simulink model "multilevelinverter1"  (R2014a)
settings: Solver=ode23tb  StartTime=0.0  StopTime=1  RelTol=1e-3
undefined symbols (not defined in the file): a, Gn, Ipvn, Iscn, k, Ki, Kv, Npp, Ns, Nss, q, Rp, Rs, Tn, Vocn
libraries: powerlib x102, simulink x34, dsparch4 x12, powerlib_extras x12, powerlib_meascontrol x3
(part 1 of 2)
settings Model: Creator=Muruganandham  LastModifiedBy=selva
settings DataIOCC: SignalLoggingSaveFormat=ModelDataLogs
settings OptimizationCC: ExpressionDepthLimit=2147483647
settings DebuggingCC: UnderspecifiedInitializationDetection=Classic  FcnCallInpInsideContextMsg=UseLocalSettings  StateNameClashWarn=warning
settings GRTTargetCC: CombineOutputUpdateFcns=off  GRTInterface=on

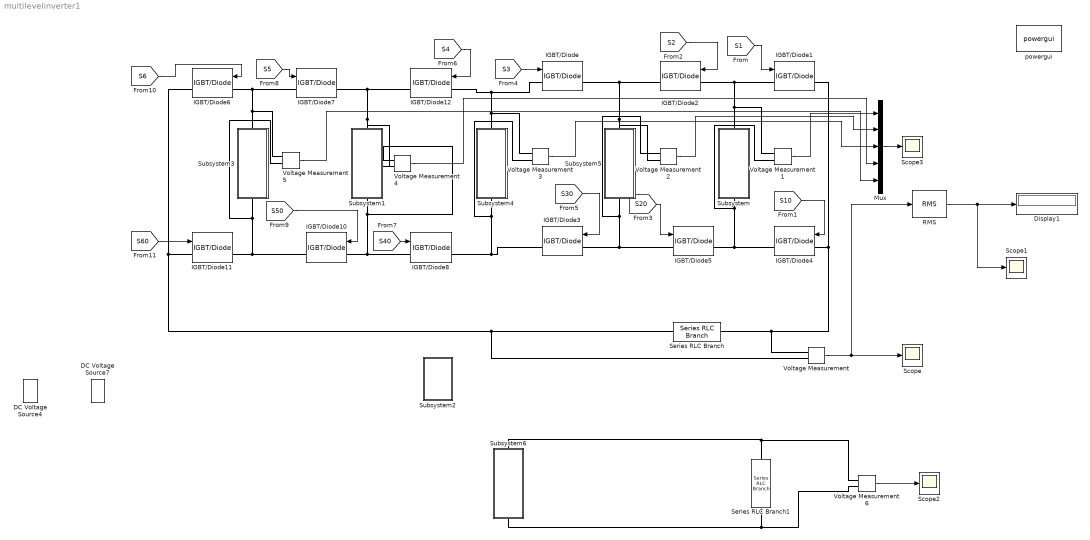
== system multilevelinverter1 ==
  DC Voltage Source4 : powerlib/Electrical Sources/DC Voltage Source  Amplitude=100  Measurements=None
  DC Voltage Source7 : powerlib/Electrical Sources/DC Voltage Source  Amplitude=100  Measurements=None
  Display1 : Display
  IGBT/Diode{,1..8,10..12} (12 alike) : powerlib/Power Electronics/IGBT//Diode  Ron=1e-3  Rs=1e5  Cs=inf  Measurements=on
  Mux : Mux  Inputs=5
  RMS : powerlib_meascontrol/Measurements/RMS  TrueRMS=on  Freq=50  RMSInit=0  Ts=0
  Scope{,1..3} (4 alike) : Scope
      Scope settings: YMin=-300  YMax=300  SaveName=bh
      Scope1 settings: YMin=0  YMax=400  SaveName=bh1
      Scope2 settings: YMin=31.5  YMax=33  SaveName=bh2
      Scope3 settings: YMin=-400  YMax=400  SaveName=bh3
  Series RLC Branch : powerlib/Elements/Series RLC Branch  LConnTagsString=__new0  RConnTagsString=__new0  BranchType=R  Resistance=50  Inductance=1e-3  SetiL0=off  InitialCurrent=0  Capacitance=1e-6  Setx0=off  InitialVoltage=0  Measurements=None
  Series RLC Branch1 : powerlib/Elements/Series RLC Branch  LConnTagsString=__new0  RConnTagsString=__new0  BranchType=R  Resistance=50  Inductance=1e-3  SetiL0=off  InitialCurrent=0  Capacitance=1e-6  Setx0=off  InitialVoltage=0  Measurements=None
  Subsystem : Subsystem
  Subsystem1 : Subsystem
  Subsystem2 : Subsystem  mask{fc=5e3, m=1}
      mask prompts: fc "Switching frequency"; m "modulation index"
  Subsystem3 : Subsystem
  Subsystem4 : Subsystem
  Subsystem5 : Subsystem
  Subsystem6 : Subsystem
  Voltage Measurement{,1..6} (7 alike) : powerlib/Measurements/Voltage Measurement  PhasorSimulation=off  OutputType=Complex  PSBequivalent=0
  powergui : powerlib/powergui  Priority=1  SimulationMode=Discrete  SolverType=Tustin  SampleTime=50e-5  frequency=60  SPID=off  DisableSnubberDevices=off  DisableRonSwitches=off  DisableVfSwitches=off  SwTol=0  Interpol=off  DisplayEquations=off  Ts=0  methode=off  frequencyindice=0  Pbase=100e6  ErrMax=1e-4  Iterations=50  UnitsV=kV  UnitsW=MW  FunctionMessages=off  echomessages=off  HookPort=off  EnableUseOfTLC=off  x0status=blocks  RestoreLinks=warning  ResistiveCurrentMeasurement=off  Frange=[0:2:500]  Ylog=off  Xlog=on  ShowGrid=off  save=off  variable=ZData  structure=bh  ZoomFFT=off  StartTime=0.0  cycles=50  DisplayStyle=1  fundamental=50  FreqAxis=off  MaxFrequency=1000  frequencyindicesteady=1  RmsSteady=1  display=off
  wires:
  [S1] -> IGBT/Diode1/1
  [S10] -> IGBT/Diode4/1
  [S2] -> IGBT/Diode2/1
  [S20] -> IGBT/Diode5/1
  [S3] -> IGBT/Diode/1
  [S30] -> IGBT/Diode3/1
  Voltage Measurement/1 -> RMS/1, Scope/1
  [S40] -> IGBT/Diode8/1
  [S6] -> IGBT/Diode6/1
  [S4] -> IGBT/Diode12/1
  [S5] -> IGBT/Diode7/1
  [S50] -> IGBT/Diode10/1
  [S60] -> IGBT/Diode11/1
  RMS/1 -> Scope1/1, Display1/1
  Voltage Measurement2/1 -> Mux/2
  Voltage Measurement1/1 -> Mux/1
  Voltage Measurement3/1 -> Mux/3
  Voltage Measurement4/1 -> Mux/4
  Voltage Measurement5/1 -> Mux/5
  Mux/1 -> Scope3/1
  Voltage Measurement6/1 -> Scope2/1
  connections:
  IGBT/Diode2/RConn1 -- IGBT/Diode/RConn1 -- Voltage Measurement2/LConn2 -- Subsystem5/RConn1
  IGBT/Diode2/LConn1 -- Voltage Measurement1/LConn1 -- Subsystem/LConn1 -- IGBT/Diode1/LConn1
  IGBT/Diode5/LConn1 -- Voltage Measurement2/LConn1 -- Subsystem5/LConn1 -- IGBT/Diode3/LConn1
  IGBT/Diode5/RConn1 -- Voltage Measurement1/LConn2 -- Subsystem/RConn1 -- IGBT/Diode4/RConn1
  Series RLC Branch/RConn1 -- IGBT/Diode1/RConn1 -- IGBT/Diode4/LConn1 -- Voltage Measurement/LConn1
  IGBT/Diode6/LConn1 -- Voltage Measurement5/LConn1 -- Subsystem3/LConn1 -- IGBT/Diode7/LConn1
  IGBT/Diode7/RConn1 -- Voltage Measurement4/LConn2 -- Subsystem1/RConn1 -- IGBT/Diode12/RConn1
  IGBT/Diode11/RConn1 -- Voltage Measurement5/LConn2 -- Subsystem3/RConn1 -- IGBT/Diode10/RConn1
  IGBT/Diode10/LConn1 -- Voltage Measurement4/LConn1 -- Subsystem1/LConn1 -- IGBT/Diode8/LConn1
  Series RLC Branch/LConn1 -- Voltage Measurement/LConn2 -- IGBT/Diode11/LConn1 -- IGBT/Diode6/RConn1
  IGBT/Diode/LConn1 -- Voltage Measurement3/LConn1 -- Subsystem4/LConn1 -- IGBT/Diode12/LConn1
  IGBT/Diode3/RConn1 -- Voltage Measurement3/LConn2 -- Subsystem4/RConn1 -- IGBT/Diode8/RConn1
  Series RLC Branch1/RConn1 -- Voltage Measurement6/LConn1 -- Subsystem6/LConn1
  Subsystem6/RConn1 -- Voltage Measurement6/LConn2 -- Series RLC Branch1/LConn1

== system multilevelinverter1/Subsystem ==
  Current Measurement : powerlib/Measurements/Current Measurement  PhasorSimulation=off  OutputType=Complex  PSBequivalent=0
  Divide : Product  Inputs=**
  Irradiation [W/m2] 1 : Constant  Value=1000
  Irradiation [W/m2] 2 : Constant
  PV Boost Converter1 : Subsystem
  PV model subsystem1 : Subsystem
  Temperature [K]1 : Constant  Value=25+273.15
  + : PMIOPort  Port=1  Side=Left
  - : PMIOPort  Port=2  Side=Right
  wires:
  Temperature [K]1/1 -> PV model subsystem1/1(T)
  Divide/1 -> PV model subsystem1/2(G)
  Irradiation [W/m2] 1/1 -> Divide/1
  Irradiation [W/m2] 2/1 -> Divide/2
  connections:
  PV Boost Converter1/LConn2 -- PV model subsystem1/RConn2
  Current Measurement/LConn1 -- PV model subsystem1/RConn1
  PV Boost Converter1/LConn1 -- Current Measurement/RConn1
  PV Boost Converter1/RConn1 -- +/RConn1
  PV Boost Converter1/RConn2 -- -/RConn1

== system multilevelinverter1/Subsystem1 ==
  Current Measurement : powerlib/Measurements/Current Measurement  PhasorSimulation=off  OutputType=Complex  PSBequivalent=0
  Divide : Product  Inputs=**
  Irradiation [W/m2] 1 : Constant  Value=1000
  Irradiation [W/m2] 2 : Constant
  PV Boost Converter1 : Subsystem
  PV model subsystem1 : Subsystem
  Temperature [K]1 : Constant  Value=25+273.15
  + : PMIOPort  Port=1  Side=Left
  - : PMIOPort  Port=2  Side=Right
  wires:
  Irradiation [W/m2] 2/1 -> Divide/2
  Irradiation [W/m2] 1/1 -> Divide/1
  Divide/1 -> PV model subsystem1/2(G)
  Temperature [K]1/1 -> PV model subsystem1/1(T)
  connections:
  PV Boost Converter1/RConn2 -- -/RConn1
  PV Boost Converter1/RConn1 -- +/RConn1
  PV Boost Converter1/LConn1 -- Current Measurement/RConn1
  Current Measurement/LConn1 -- PV model subsystem1/RConn1
  PV Boost Converter1/LConn2 -- PV model subsystem1/RConn2

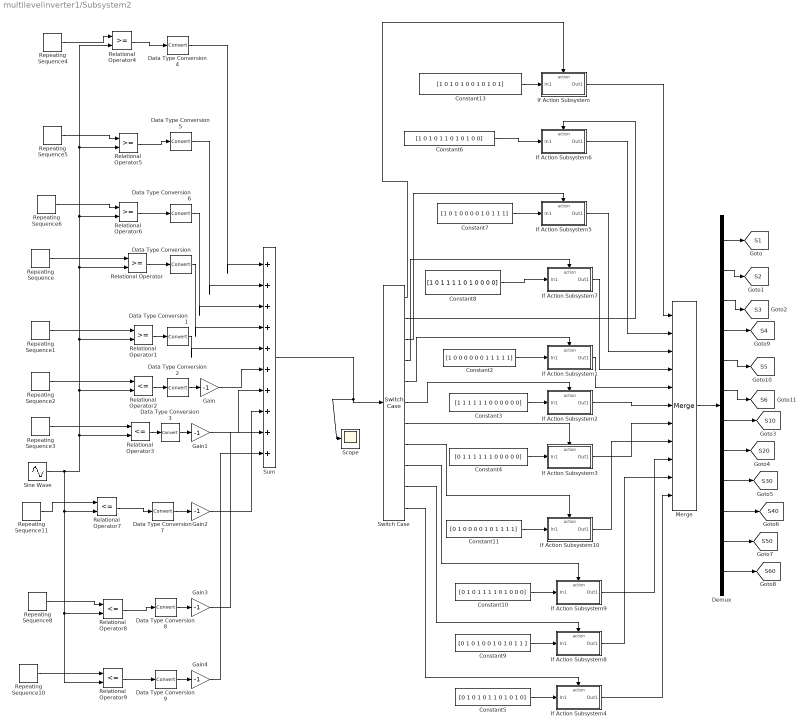
== system multilevelinverter1/Subsystem2 ==
  Constant10 : Constant  Value=[0 1 0 1 1 1 1 0 1 0 0 0]
  Constant11 : Constant  Value=[0 1 0 0 0 0 1 0 1 1 1 1]
  Constant13 : Constant  Value=[1 0 1 0 1 0 0 1 0 1 0 1]
  Constant2 : Constant  Value=[1 0 0 0 0 0 0 1 1 1 1 1]
  Constant3 : Constant  Value=[1 1 1 1 1 1 0 0 0 0 0 0]
  Constant4 : Constant  Value=[0 1 1 1 1 1 1 0 0 0 0 0]
  Constant5 : Constant  Value=[0 1 0 1 0 1 1 0 1 0 1 0]
  Constant6 : Constant  Value=[1 0 1 0 1 1 0 1 0 1 0 0]
  Constant7 : Constant  Value=[1 0 1 0 0 0 0 1 0 1 1 1]
  Constant8 : Constant  Value=[1 0 1 1 1 1 0 1 0 0 0 0]
  Constant9 : Constant  Value=[0 1 0 1 0 0 1 0 1 0 1 1 ]
  Data Type Conversion{,1..9} (10 alike) : DataTypeConversion
  Demux : Demux  Outputs=12
  Gain{,1..4} (5 alike) : Gain  Gain=-1
  If Action Subsystem : Subsystem  TreatAsAtomicUnit=on
  If Action Subsystem1 : Subsystem  TreatAsAtomicUnit=on
  If Action Subsystem10 : Subsystem  TreatAsAtomicUnit=on
  If Action Subsystem2 : Subsystem  TreatAsAtomicUnit=on
  If Action Subsystem3 : Subsystem  TreatAsAtomicUnit=on
  If Action Subsystem4 : Subsystem  TreatAsAtomicUnit=on
  If Action Subsystem5 : Subsystem  TreatAsAtomicUnit=on
  If Action Subsystem6 : Subsystem  TreatAsAtomicUnit=on
  If Action Subsystem7 : Subsystem  TreatAsAtomicUnit=on
  If Action Subsystem8 : Subsystem  TreatAsAtomicUnit=on
  If Action Subsystem9 : Subsystem  TreatAsAtomicUnit=on
  Merge : Merge  Inputs=11
  Relational Operator{,1,4..6} (5 alike) : RelationalOperator  OutDataTypeStr=boolean
  Relational Operator{2..3,7..9} (5 alike) : RelationalOperator  Operator=<=  OutDataTypeStr=boolean
  Repeating Sequence : simulink/Sources/Repeating Sequence  rep_seq_t="[0 (1/fc)/2  (1/fc)]"  rep_seq_y=[2 1 2]
  Repeating Sequence1 : simulink/Sources/Repeating Sequence  rep_seq_t="[0 (1/fc)/2  (1/fc)]"  rep_seq_y=[1 0 1]
  Repeating Sequence10 : simulink/Sources/Repeating Sequence  rep_seq_t="[0 (1/fc)/2  (1/fc)]"  rep_seq_y=[-5 -4 -5]
  Repeating Sequence11 : simulink/Sources/Repeating Sequence  rep_seq_t="[0 (1/fc)/2  (1/fc)]"  rep_seq_y=[-3 -2 -3]
  Repeating Sequence2 : simulink/Sources/Repeating Sequence  rep_seq_t="[0 (1/fc)/2  (1/fc)]"  rep_seq_y=[-1 0 -1]
  Repeating Sequence3 : simulink/Sources/Repeating Sequence  rep_seq_t="[0 (1/fc)/2  (1/fc)]"  rep_seq_y=[-2 -1 -2]
  Repeating Sequence4 : simulink/Sources/Repeating Sequence  rep_seq_t="[0 (1/fc)/2  (1/fc)]"  rep_seq_y=[4 5 4]
  Repeating Sequence5 : simulink/Sources/Repeating Sequence  rep_seq_t="[0 (1/fc)/2  (1/fc)]"  rep_seq_y=[4 3 4]
  Repeating Sequence6 : simulink/Sources/Repeating Sequence  rep_seq_t="[0 (1/fc)/2  (1/fc)]"  rep_seq_y=[3 2 3]
  Repeating Sequence8 : simulink/Sources/Repeating Sequence  rep_seq_t="[0 (1/fc)/2  (1/fc)]"  rep_seq_y=[-4 -3 -4]
  Scope : Scope
  Sine Wave : Sin  Amplitude=6*m  Frequency=2*pi*50  SampleTime=0
  Sum : Sum  Inputs=|++++++++++
  Switch Case : SwitchCase  CaseConditions={-5, -4, -3, -2, -1, 0, 1, 2, 3, 4, 5}  ShowDefaultCase=off
  tag scope: S10=global, S1=global, S20=global, S2=global, S30=global, S3=global, S40=global, S4=global, S50=global, S5=global, S60=global, S6=global
  wires:
  Data Type Conversion3/1 -> Gain1/1
  Data Type Conversion2/1 -> Gain/1
  Relational Operator3/1 -> Data Type Conversion3/1
  Relational Operator2/1 -> Data Type Conversion2/1
  Repeating Sequence3/1 -> Relational Operator3/1
  Repeating Sequence2/1 -> Relational Operator2/1
  Repeating Sequence1/1 -> Relational Operator1/1
  Repeating Sequence/1 -> Relational Operator/1
  Relational Operator1/1 -> Data Type Conversion1/1
  Relational Operator/1 -> Data Type Conversion/1
  Merge/1 -> Demux/1
  If Action Subsystem/1(Out1) -> Merge/1
  Constant4/1 -> If Action Subsystem3/1(In1)
  Constant3/1 -> If Action Subsystem2/1(In1)
  Constant2/1 -> If Action Subsystem1/1(In1)
  Repeating Sequence6/1 -> Relational Operator6/1
  Repeating Sequence5/1 -> Relational Operator5/1
  Repeating Sequence4/1 -> Relational Operator4/1
  Relational Operator6/1 -> Data Type Conversion6/1
  Relational Operator5/1 -> Data Type Conversion5/1
  Relational Operator4/1 -> Data Type Conversion4/1
  Repeating Sequence8/1 -> Relational Operator8/1
  Repeating Sequence11/1 -> Relational Operator7/1
  Sine Wave/1 -> Relational Operator9/2, Relational Operator8/2, Relational Operator7/2, Relational Operator3/2, Relational Operator2/2, Relational Operator6/2, Relational Operator5/2, Relational Operator4/2, Relational Operator/2, Relational Operator1/2
  Relational Operator9/1 -> Data Type Conversion9/1
  Relational Operator8/1 -> Data Type Conversion8/1
  Relational Operator7/1 -> Data Type Conversion7/1
  Data Type Conversion9/1 -> Gain4/1
  Data Type Conversion8/1 -> Gain3/1
  Data Type Conversion7/1 -> Gain2/1
  Repeating Sequence10/1 -> Relational Operator9/1
  Data Type Conversion4/1 -> Sum/1
  Data Type Conversion5/1 -> Sum/2
  Data Type Conversion6/1 -> Sum/3
  Data Type Conversion/1 -> Sum/4
  Data Type Conversion1/1 -> Sum/5
  Gain/1 -> Sum/6
  Gain1/1 -> Sum/7
  Gain2/1 -> Sum/8
  Gain3/1 -> Sum/9
  Gain4/1 -> Sum/10
  Switch Case/6 -> If Action Subsystem2/Action
  If Action Subsystem6/1(Out1) -> Merge/2
  If Action Subsystem5/1(Out1) -> Merge/3
  If Action Subsystem7/1(Out1) -> Merge/4
  If Action Subsystem1/1(Out1) -> Merge/5
  If Action Subsystem2/1(Out1) -> Merge/6
  If Action Subsystem3/1(Out1) -> Merge/7
  Constant9/1 -> If Action Subsystem8/1(In1)
  Constant10/1 -> If Action Subsystem9/1(In1)
  Constant11/1 -> If Action Subsystem10/1(In1)
  Switch Case/11 -> If Action Subsystem4/Action
  If Action Subsystem4/1(Out1) -> Merge/11
  Switch Case/10 -> If Action Subsystem8/Action
  Switch Case/9 -> If Action Subsystem9/Action
  Switch Case/8 -> If Action Subsystem10/Action
  Switch Case/7 -> If Action Subsystem3/Action
  Switch Case/5 -> If Action Subsystem1/Action
  Switch Case/4 -> If Action Subsystem7/Action
  Switch Case/3 -> If Action Subsystem5/Action
  Switch Case/2 -> If Action Subsystem6/Action
  Switch Case/1 -> If Action Subsystem/Action
  Constant6/1 -> If Action Subsystem6/1(In1)
  Constant7/1 -> If Action Subsystem5/1(In1)
  Constant8/1 -> If Action Subsystem7/1(In1)
  If Action Subsystem10/1(Out1) -> Merge/8
  If Action Subsystem9/1(Out1) -> Merge/9
  If Action Subsystem8/1(Out1) -> Merge/10
  Demux/3 -> [S3]
  Demux/2 -> [S2]
  Demux/1 -> [S1]
  Demux/7 -> [S10]
  Demux/8 -> [S20]
  Demux/9 -> [S30]
  Demux/10 -> [S40]
  Demux/11 -> [S50]
  Demux/12 -> [S60]
  Demux/6 -> [S6]
  Demux/5 -> [S5]
  Demux/4 -> [S4]
  Sum/1 -> Scope/1, Switch Case/1
  Constant5/1 -> If Action Subsystem4/1(In1)
  Constant13/1 -> If Action Subsystem/1(In1)

== system multilevelinverter1/Subsystem3 ==
  Current Measurement : powerlib/Measurements/Current Measurement  PhasorSimulation=off  OutputType=Complex  PSBequivalent=0
  Divide : Product  Inputs=**
  Irradiation [W/m2] 1 : Constant  Value=1000
  Irradiation [W/m2] 2 : Constant
  PV Boost Converter1 : Subsystem
  PV model subsystem1 : Subsystem
  Temperature [K]1 : Constant  Value=25+273.15
  + : PMIOPort  Port=1  Side=Left
  - : PMIOPort  Port=2  Side=Right
  wires:
  Irradiation [W/m2] 2/1 -> Divide/2
  Irradiation [W/m2] 1/1 -> Divide/1
  Divide/1 -> PV model subsystem1/2(G)
  Temperature [K]1/1 -> PV model subsystem1/1(T)
  connections:
  PV Boost Converter1/RConn2 -- -/RConn1
  PV Boost Converter1/RConn1 -- +/RConn1
  PV Boost Converter1/LConn1 -- Current Measurement/RConn1
  Current Measurement/LConn1 -- PV model subsystem1/RConn1
  PV Boost Converter1/LConn2 -- PV model subsystem1/RConn2

== system multilevelinverter1/Subsystem4 ==
  Current Measurement : powerlib/Measurements/Current Measurement  PhasorSimulation=off  OutputType=Complex  PSBequivalent=0
  Divide : Product  Inputs=**
  Irradiation [W/m2] 1 : Constant  Value=1000
  Irradiation [W/m2] 2 : Constant
  PV Boost Converter1 : Subsystem
  PV model subsystem1 : Subsystem
  Temperature [K]1 : Constant  Value=25+273.15
  + : PMIOPort  Port=1  Side=Left
  - : PMIOPort  Port=2  Side=Right
  wires:
  Irradiation [W/m2] 2/1 -> Divide/2
  Irradiation [W/m2] 1/1 -> Divide/1
  Divide/1 -> PV model subsystem1/2(G)
  Temperature [K]1/1 -> PV model subsystem1/1(T)
  connections:
  PV Boost Converter1/RConn2 -- -/RConn1
  PV Boost Converter1/RConn1 -- +/RConn1
  PV Boost Converter1/LConn1 -- Current Measurement/RConn1
  Current Measurement/LConn1 -- PV model subsystem1/RConn1
  PV Boost Converter1/LConn2 -- PV model subsystem1/RConn2

== system multilevelinverter1/Subsystem5 ==
  Current Measurement : powerlib/Measurements/Current Measurement  PhasorSimulation=off  OutputType=Complex  PSBequivalent=0
  Divide : Product  Inputs=**
  Irradiation [W/m2] 1 : Constant  Value=1000
  Irradiation [W/m2] 2 : Constant
  PV Boost Converter1 : Subsystem
  PV model subsystem1 : Subsystem
  Temperature [K]1 : Constant  Value=25+273.15
  + : PMIOPort  Port=1  Side=Left
  - : PMIOPort  Port=2  Side=Right
  wires:
  Temperature [K]1/1 -> PV model subsystem1/1(T)
  Divide/1 -> PV model subsystem1/2(G)
  Irradiation [W/m2] 1/1 -> Divide/1
  Irradiation [W/m2] 2/1 -> Divide/2
  connections:
  PV Boost Converter1/LConn2 -- PV model subsystem1/RConn2
  Current Measurement/LConn1 -- PV model subsystem1/RConn1
  PV Boost Converter1/LConn1 -- Current Measurement/RConn1
  PV Boost Converter1/RConn1 -- +/RConn1
  PV Boost Converter1/RConn2 -- -/RConn1

== system multilevelinverter1/Subsystem6 ==
  Current Measurement : powerlib/Measurements/Current Measurement  PhasorSimulation=off  OutputType=Complex  PSBequivalent=0
  Divide : Product  Inputs=**
  Irradiation [W/m2] 1 : Constant  Value=1000
  Irradiation [W/m2] 2 : Constant
  PV Boost Converter1 : Subsystem
  PV model subsystem1 : Subsystem
  Temperature [K]1 : Constant  Value=25+273.15
  + : PMIOPort  Port=1  Side=Left
  - : PMIOPort  Port=2  Side=Right
  wires:
  Temperature [K]1/1 -> PV model subsystem1/1(T)
  Divide/1 -> PV model subsystem1/2(G)
  Irradiation [W/m2] 1/1 -> Divide/1
  Irradiation [W/m2] 2/1 -> Divide/2
  connections:
  PV Boost Converter1/LConn2 -- PV model subsystem1/RConn2
  Current Measurement/LConn1 -- PV model subsystem1/RConn1
  PV Boost Converter1/LConn1 -- Current Measurement/RConn1
  PV Boost Converter1/RConn1 -- +/RConn1
  PV Boost Converter1/RConn2 -- -/RConn1

== system multilevelinverter1/Subsystem/PV Boost Converter1 ==
  Analog Filter Design : dsparch4/Analog Filter Design  method=Butterworth  filttype=Lowpass  N=8  Wlo=30  Whi=80  Rp=2  Rs=40
  Analog Filter Design1 : dsparch4/Analog Filter Design  method=Butterworth  filttype=Lowpass  N=8  Wlo=30  Whi=80  Rp=2  Rs=40
  Current Measurement : powerlib/Measurements/Current Measurement  PhasorSimulation=off  OutputType=Complex  PSBequivalent=0
  Diode : powerlib/Power Electronics/Diode  Ron=0.001  Lon=0  Vf=0.8  IC=0  UseSnubber=off  Rs=500  Cs=250e-9  Measurements=on
  MPPT : Subsystem
  Mosfet : powerlib/Power Electronics/Mosfet  Ron=0.1  Lon=0  Rd=0.01  Vfd=0  IC=0  Rs=1e5  Cs=inf  Measurements=on
  PI CONTOLER : Subsystem
  Relational Operator1 : RelationalOperator  Operator=<=  OutDataTypeStr=boolean
  Repeating Sequence : simulink/Sources/Repeating Sequence  rep_seq_t=[0 0.0001 0.0002]  rep_seq_y=[0 10 0]
  Scope{1..3,8} (4 alike) : Scope
      Scope1 settings: SaveName=ScopeData2
      Scope2 settings: SaveName=ScopeData3
      Scope3 settings: YMin=-20  YMax=100  SaveName=ScopeData12
      Scope8 settings: YMin=31.943  YMax=31.943  SaveName=ScopeData4
  Series RLC Branch : powerlib/Elements/Series RLC Branch  LConnTagsString=__new0  RConnTagsString=__new0  BranchType=L  Resistance=1  Inductance=1e-3  SetiL0=off  InitialCurrent=0  Capacitance=1e-6  Setx0=off  InitialVoltage=0  Measurements=None
  Series RLC Branch1 : powerlib/Elements/Series RLC Branch  LConnTagsString=__new0  RConnTagsString=__new0  BranchType=C  Resistance=1  Inductance=12e-3  SetiL0=off  InitialCurrent=0  Capacitance=2200e-6  Setx0=off  InitialVoltage=0  Measurements=None
  Voltage Measurement1 : powerlib/Measurements/Voltage Measurement  PhasorSimulation=off  OutputType=Complex  PSBequivalent=0
  Voltage Measurement2 : powerlib/Measurements/Voltage Measurement  PhasorSimulation=off  OutputType=Complex  PSBequivalent=0
  + : PMIOPort  Port=1  Side=Right
  - : PMIOPort  Port=2  Side=Right
  Vpv+ : PMIOPort  Tag=PMCPort  Port=3  Side=Left
  Vpv- : PMIOPort  Tag=PMCPort  Port=4  Side=Left
  wires:
  Analog Filter Design1/1 -> MPPT/1(V)
  Analog Filter Design/1 -> MPPT/2(I)
  MPPT/1(D) -> Relational Operator1/2
  Relational Operator1/1 -> Scope1/1
  Repeating Sequence/1 -> Scope2/1, Relational Operator1/1
  Current Measurement/1 -> Analog Filter Design/1
  Voltage Measurement1/1 -> Scope8/1, [A1]
  [A1] -> PI CONTOLER/1(In1)
  PI CONTOLER/1(Out1) -> [G]
  Voltage Measurement2/1 -> Scope3/1, Analog Filter Design1/1
  [G] -> Mosfet/1
  connections:
  Current Measurement/LConn1 -- Vpv+/RConn1
  Diode/RConn1 -- Voltage Measurement1/LConn1 -- +/RConn1 -- Series RLC Branch1/LConn1
  Series RLC Branch/LConn1 -- Current Measurement/RConn1 -- Voltage Measurement2/LConn1
  Series RLC Branch1/RConn1 -- Voltage Measurement1/LConn2 -- -/RConn1 -- Mosfet/RConn1 -- Voltage Measurement2/LConn2 -- Vpv-/RConn1
  Diode/LConn1 -- Mosfet/LConn1 -- Series RLC Branch/RConn1

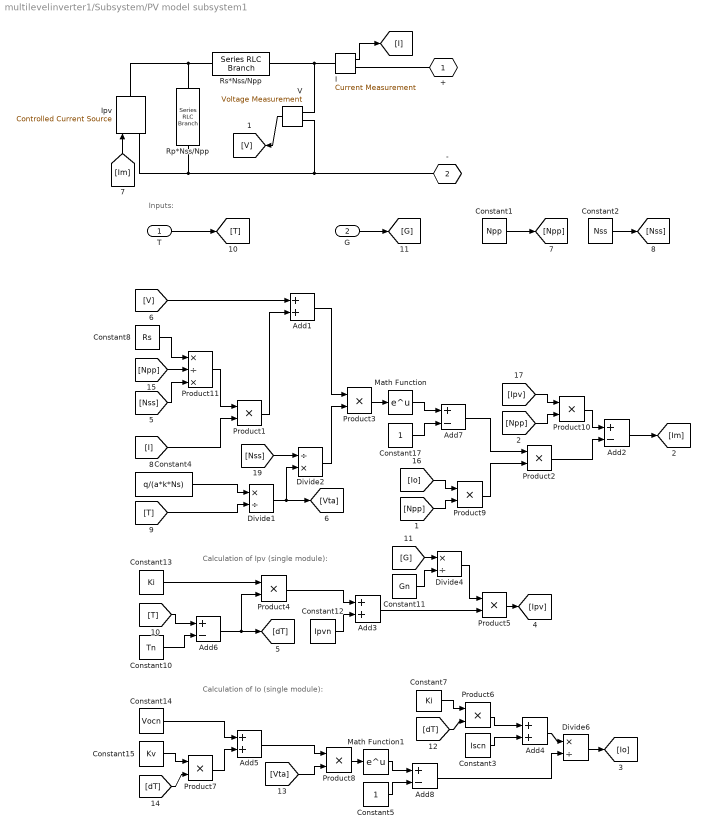
== system multilevelinverter1/Subsystem/PV model subsystem1 ==
  note: Inputs:
  note: Calculation of Ipv (single module):
  note: Calculation of Io (single module):
  T : Inport
  G : Inport  Port=2
  Add{1,3..5} (4 alike) : Sum
  Add{2,6..8} (4 alike) : Sum  Inputs=+-
  Constant1 : Constant  Value=Npp
  Constant10 : Constant  Value=Tn
  Constant11 : Constant  Value=Gn
  Constant12 : Constant  Value=Ipvn
  Constant13 : Constant  Value=Ki
  Constant14 : Constant  Value=Vocn
  Constant15 : Constant  Value=Kv
  Constant17 : Constant
  Constant2 : Constant  Value=Nss
  Constant3 : Constant  Value=Iscn
  Constant4 : Constant  Value=q/(a*k*Ns)
  Constant5 : Constant
  Constant7 : Constant  Value=Ki
  Constant8 : Constant  Value=Rs
  Divide1 : Product  Inputs=*/
  Divide2 : Product  Inputs=/*
  Divide4 : Product  Inputs=*/
  Divide6 : Product  Inputs=*/
  I : powerlib/Measurements/Current Measurement  PhasorSimulation=off  OutputType=Complex  PSBequivalent=0
  Ipv : powerlib/Electrical Sources/Controlled Current Source  Initialize=on  Source_Type=DC  Amplitude=00  Phase=0  Frequency=0  Measurements=None
  Math Function : Math  SaturateOnIntegerOverflow=on
  Math Function1 : Math  SaturateOnIntegerOverflow=on
  Product{1..10} (10 alike) : Product  RndMeth=Zero
  Product11 : Product  Inputs=*/*  RndMeth=Zero
  Rp*Nss/Npp : powerlib/Elements/Series RLC Branch  LConnTagsString=__new0  RConnTagsString=__new0  BranchType=R  Resistance=Rp*Nss/Npp  Inductance=1e-3  SetiL0=off  InitialCurrent=0  Capacitance=1e-6  Setx0=off  InitialVoltage=0  Measurements=None
  Rs*Nss/Npp : powerlib/Elements/Series RLC Branch  LConnTagsString=__new0  RConnTagsString=__new0  BranchType=R  Resistance=Rs*Nss/Npp  Inductance=1e-3  SetiL0=off  InitialCurrent=0  Capacitance=1e-6  Setx0=off  InitialVoltage=0  Measurements=None
  "V " : powerlib/Measurements/Voltage Measurement  PhasorSimulation=off  OutputType=Complex  PSBequivalent=0
  + : PMIOPort  Port=1  Side=Right
  - : PMIOPort  Port=2  Side=Right
  wires:
  I/1 -> [I]
  "V "/1 -> [V]
  [Im] -> Ipv/1
  G/1 -> [G]
  T/1 -> [T]
  Constant10/1 -> Add6/2
  [T] -> Add6/1
  [I] -> Product1/2
  Constant4/1 -> Divide1/1
  [T] -> Divide1/2
  [V] -> Add1/1
  Product3/1 -> Math Function/1
  Add2/1 -> [Im]
  Add1/1 -> Product3/1
  [G] -> Divide4/1
  Constant11/1 -> Divide4/2
  Constant13/1 -> Product4/1
  [dT] -> Product6/2
  Constant7/1 -> Product6/1
  [dT] -> Product7/2
  Constant14/1 -> Add5/1
  Product8/1 -> Math Function1/1
  Add5/1 -> Product8/1
  Constant17/1 -> Add7/2
  Add7/1 -> Product2/1
  Constant5/1 -> Add8/2
  Math Function1/1 -> Add8/1
  Divide6/1 -> [Io]
  Product5/1 -> [Ipv]
  Product1/1 -> Add1/2
  Math Function/1 -> Add7/1
  Product4/1 -> Add3/1
  Add3/1 -> Product5/2
  Divide4/1 -> Product5/1
  Product7/1 -> Add5/2
  Constant15/1 -> Product7/1
  [Vta] -> Product8/2
  Add8/1 -> Divide6/2
  Constant3/1 -> Add4/2
  Product6/1 -> Add4/1
  Constant12/1 -> Add3/2
  Product2/1 -> Add2/2
  Product9/1 -> Product2/2
  [Io] -> Product9/1
  [Npp] -> Product9/2
  Constant1/1 -> [Npp]
  Constant2/1 -> [Nss]
  [Ipv] -> Product10/1
  [Npp] -> Product10/2
  Product10/1 -> Add2/1
  Constant8/1 -> Product11/1
  [Npp] -> Product11/2
  [Nss] -> Product11/3
  Product11/1 -> Product1/1
  [Nss] -> Divide2/1
  Divide1/1 -> Divide2/2, [Vta]
  Divide2/1 -> Product3/2
  Add6/1 -> [dT], Product4/2
  Add4/1 -> Divide6/1
  connections:
  I/LConn1 -- "V "/LConn1 -- Rs*Nss/Npp/RConn1
  -/RConn1 -- Rp*Nss/Npp/RConn1 -- Ipv/LConn1 -- "V "/LConn2
  Ipv/RConn1 -- Rs*Nss/Npp/LConn1 -- Rp*Nss/Npp/LConn1
  +/RConn1 -- I/RConn1

== system multilevelinverter1/Subsystem1/PV Boost Converter1 ==
  Analog Filter Design : dsparch4/Analog Filter Design  method=Butterworth  filttype=Lowpass  N=8  Wlo=30  Whi=80  Rp=2  Rs=40
  Analog Filter Design1 : dsparch4/Analog Filter Design  method=Butterworth  filttype=Lowpass  N=8  Wlo=30  Whi=80  Rp=2  Rs=40
  Current Measurement : powerlib/Measurements/Current Measurement  PhasorSimulation=off  OutputType=Complex  PSBequivalent=0
  Diode : powerlib/Power Electronics/Diode  Ron=0.001  Lon=0  Vf=0.8  IC=0  UseSnubber=off  Rs=500  Cs=250e-9  Measurements=on
  MPPT : Subsystem
  Mosfet : powerlib/Power Electronics/Mosfet  Ron=0.1  Lon=0  Rd=0.01  Vfd=0  IC=0  Rs=1e5  Cs=inf  Measurements=on
  PI CONTOLER : Subsystem
  Relational Operator1 : RelationalOperator  Operator=<=  OutDataTypeStr=boolean
  Repeating Sequence : simulink/Sources/Repeating Sequence  rep_seq_t=[0 0.0001 0.0002]  rep_seq_y=[0 10 0]
  Scope{1..3,8} (4 alike) : Scope
      Scope1 settings: SaveName=ScopeData2
      Scope2 settings: SaveName=ScopeData3
      Scope3 settings: YMin=-20  YMax=100  SaveName=ScopeData12
      Scope8 settings: YMin=31.943  YMax=31.943  SaveName=ScopeData4
  Series RLC Branch : powerlib/Elements/Series RLC Branch  LConnTagsString=__new0  RConnTagsString=__new0  BranchType=L  Resistance=1  Inductance=1e-3  SetiL0=off  InitialCurrent=0  Capacitance=1e-6  Setx0=off  InitialVoltage=0  Measurements=None
  Series RLC Branch1 : powerlib/Elements/Series RLC Branch  LConnTagsString=__new0  RConnTagsString=__new0  BranchType=C  Resistance=1  Inductance=12e-3  SetiL0=off  InitialCurrent=0  Capacitance=2200e-6  Setx0=off  InitialVoltage=0  Measurements=None
  Voltage Measurement1 : powerlib/Measurements/Voltage Measurement  PhasorSimulation=off  OutputType=Complex  PSBequivalent=0
  Voltage Measurement2 : powerlib/Measurements/Voltage Measurement  PhasorSimulation=off  OutputType=Complex  PSBequivalent=0
  + : PMIOPort  Port=1  Side=Right
  - : PMIOPort  Port=2  Side=Right
  Vpv+ : PMIOPort  Tag=PMCPort  Port=3  Side=Left
  Vpv- : PMIOPort  Tag=PMCPort  Port=4  Side=Left
  wires:
  [G] -> Mosfet/1
  Voltage Measurement2/1 -> Analog Filter Design1/1, Scope3/1
  PI CONTOLER/1(Out1) -> [G]
  [A1] -> PI CONTOLER/1(In1)
  Voltage Measurement1/1 -> [A1], Scope8/1
  Current Measurement/1 -> Analog Filter Design/1
  Repeating Sequence/1 -> Relational Operator1/1, Scope2/1
  Relational Operator1/1 -> Scope1/1
  MPPT/1(D) -> Relational Operator1/2
  Analog Filter Design/1 -> MPPT/2(I)
  Analog Filter Design1/1 -> MPPT/1(V)
  connections:
  Series RLC Branch/RConn1 -- Mosfet/LConn1 -- Diode/LConn1
  Vpv-/RConn1 -- Voltage Measurement2/LConn2 -- Mosfet/RConn1 -- -/RConn1 -- Voltage Measurement1/LConn2 -- Series RLC Branch1/RConn1
  Voltage Measurement2/LConn1 -- Current Measurement/RConn1 -- Series RLC Branch/LConn1
  Series RLC Branch1/LConn1 -- +/RConn1 -- Voltage Measurement1/LConn1 -- Diode/RConn1
  Current Measurement/LConn1 -- Vpv+/RConn1

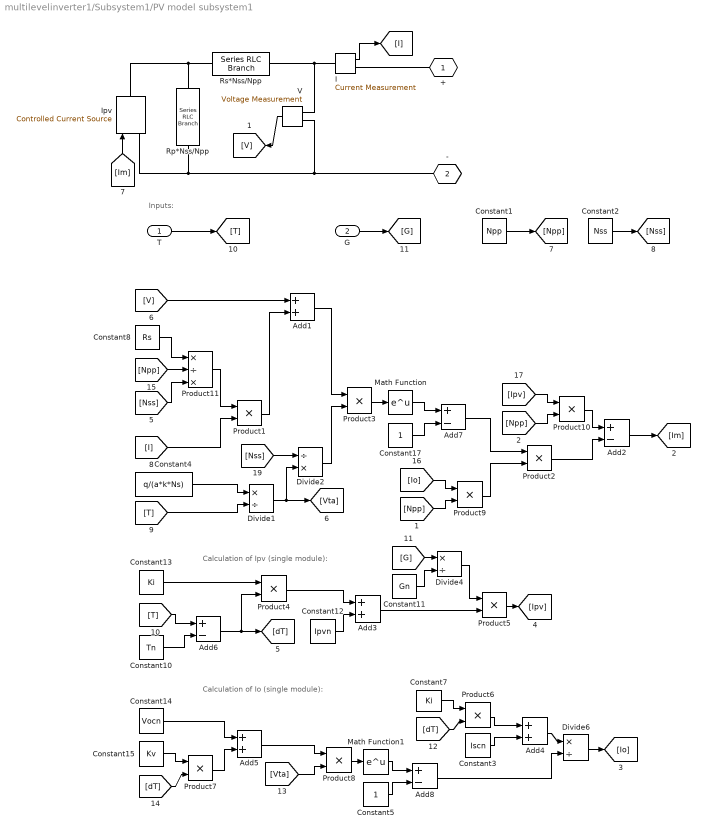
== system multilevelinverter1/Subsystem1/PV model subsystem1 ==
  note: Calculation of Io (single module):
  note: Calculation of Ipv (single module):
  note: Inputs:
  T : Inport
  G : Inport  Port=2
  Add{1,3..5} (4 alike) : Sum
  Add{2,6..8} (4 alike) : Sum  Inputs=+-
  Constant1 : Constant  Value=Npp
  Constant10 : Constant  Value=Tn
  Constant11 : Constant  Value=Gn
  Constant12 : Constant  Value=Ipvn
  Constant13 : Constant  Value=Ki
  Constant14 : Constant  Value=Vocn
  Constant15 : Constant  Value=Kv
  Constant17 : Constant
  Constant2 : Constant  Value=Nss
  Constant3 : Constant  Value=Iscn
  Constant4 : Constant  Value=q/(a*k*Ns)
  Constant5 : Constant
  Constant7 : Constant  Value=Ki
  Constant8 : Constant  Value=Rs
  Divide1 : Product  Inputs=*/
  Divide2 : Product  Inputs=/*
  Divide4 : Product  Inputs=*/
  Divide6 : Product  Inputs=*/
  I : powerlib/Measurements/Current Measurement  PhasorSimulation=off  OutputType=Complex  PSBequivalent=0
  Ipv : powerlib/Electrical Sources/Controlled Current Source  Initialize=on  Source_Type=DC  Amplitude=00  Phase=0  Frequency=0  Measurements=None
  Math Function : Math  SaturateOnIntegerOverflow=on
  Math Function1 : Math  SaturateOnIntegerOverflow=on
  Product{1..10} (10 alike) : Product  RndMeth=Zero
  Product11 : Product  Inputs=*/*  RndMeth=Zero
  Rp*Nss/Npp : powerlib/Elements/Series RLC Branch  LConnTagsString=__new0  RConnTagsString=__new0  BranchType=R  Resistance=Rp*Nss/Npp  Inductance=1e-3  SetiL0=off  InitialCurrent=0  Capacitance=1e-6  Setx0=off  InitialVoltage=0  Measurements=None
  Rs*Nss/Npp : powerlib/Elements/Series RLC Branch  LConnTagsString=__new0  RConnTagsString=__new0  BranchType=R  Resistance=Rs*Nss/Npp  Inductance=1e-3  SetiL0=off  InitialCurrent=0  Capacitance=1e-6  Setx0=off  InitialVoltage=0  Measurements=None
  "V " : powerlib/Measurements/Voltage Measurement  PhasorSimulation=off  OutputType=Complex  PSBequivalent=0
  + : PMIOPort  Port=1  Side=Right
  - : PMIOPort  Port=2  Side=Right
  wires:
  Add4/1 -> Divide6/1
  Add6/1 -> Product4/2, [dT]
  Divide2/1 -> Product3/2
  Divide1/1 -> [Vta], Divide2/2
  [Nss] -> Divide2/1
  Product11/1 -> Product1/1
  [Nss] -> Product11/3
  [Npp] -> Product11/2
  Constant8/1 -> Product11/1
  Product10/1 -> Add2/1
  [Npp] -> Product10/2
  [Ipv] -> Product10/1
  Constant2/1 -> [Nss]
  Constant1/1 -> [Npp]
  [Npp] -> Product9/2
  [Io] -> Product9/1
  Product9/1 -> Product2/2
  Product2/1 -> Add2/2
  Constant12/1 -> Add3/2
  Product6/1 -> Add4/1
  Constant3/1 -> Add4/2
  Add8/1 -> Divide6/2
  [Vta] -> Product8/2
  Constant15/1 -> Product7/1
  Product7/1 -> Add5/2
  Divide4/1 -> Product5/1
  Add3/1 -> Product5/2
  Product4/1 -> Add3/1
  Math Function/1 -> Add7/1
  Product1/1 -> Add1/2
  Product5/1 -> [Ipv]
  Divide6/1 -> [Io]
  Math Function1/1 -> Add8/1
  Constant5/1 -> Add8/2
  Add7/1 -> Product2/1
  Constant17/1 -> Add7/2
  Add5/1 -> Product8/1
  Product8/1 -> Math Function1/1
  Constant14/1 -> Add5/1
  [dT] -> Product7/2
  Constant7/1 -> Product6/1
  [dT] -> Product6/2
  Constant13/1 -> Product4/1
  Constant11/1 -> Divide4/2
  [G] -> Divide4/1
  Add1/1 -> Product3/1
  Add2/1 -> [Im]
  Product3/1 -> Math Function/1
  [V] -> Add1/1
  [T] -> Divide1/2
  Constant4/1 -> Divide1/1
  [I] -> Product1/2
  [T] -> Add6/1
  Constant10/1 -> Add6/2
  T/1 -> [T]
  G/1 -> [G]
  [Im] -> Ipv/1
  "V "/1 -> [V]
  I/1 -> [I]
  connections:
  +/RConn1 -- I/RConn1
  Rp*Nss/Npp/LConn1 -- Rs*Nss/Npp/LConn1 -- Ipv/RConn1
  "V "/LConn2 -- Ipv/LConn1 -- Rp*Nss/Npp/RConn1 -- -/RConn1
  Rs*Nss/Npp/RConn1 -- "V "/LConn1 -- I/LConn1

== system multilevelinverter1/Subsystem2/If Action Subsystem ==
  In1 : Inport
  Action Port : ActionPort  ActionType=case
  Out1 : Outport
  wires:
  In1/1 -> Out1/1

== system multilevelinverter1/Subsystem2/If Action Subsystem1 ==
  In1 : Inport
  Action Port : ActionPort  ActionType=case
  Out1 : Outport
  wires:
  In1/1 -> Out1/1

== system multilevelinverter1/Subsystem2/If Action Subsystem10 ==
  In1 : Inport
  Action Port : ActionPort  ActionType=case
  Out1 : Outport
  wires:
  In1/1 -> Out1/1

== system multilevelinverter1/Subsystem2/If Action Subsystem2 ==
  In1 : Inport
  Action Port : ActionPort  ActionType=case
  Out1 : Outport
  wires:
  In1/1 -> Out1/1

== system multilevelinverter1/Subsystem2/If Action Subsystem3 ==
  In1 : Inport
  Action Port : ActionPort  ActionType=case
  Out1 : Outport
  wires:
  In1/1 -> Out1/1

== system multilevelinverter1/Subsystem2/If Action Subsystem4 ==
  In1 : Inport
  Action Port : ActionPort  ActionType=case
  Out1 : Outport
  wires:
  In1/1 -> Out1/1

== system multilevelinverter1/Subsystem2/If Action Subsystem5 ==
  In1 : Inport
  Action Port : ActionPort  ActionType=case
  Out1 : Outport
  wires:
  In1/1 -> Out1/1

== system multilevelinverter1/Subsystem2/If Action Subsystem6 ==
  In1 : Inport
  Action Port : ActionPort  ActionType=case
  Out1 : Outport
  wires:
  In1/1 -> Out1/1

== system multilevelinverter1/Subsystem2/If Action Subsystem7 ==
  In1 : Inport
  Action Port : ActionPort  ActionType=case
  Out1 : Outport
  wires:
  In1/1 -> Out1/1

== system multilevelinverter1/Subsystem2/If Action Subsystem8 ==
  In1 : Inport
  Action Port : ActionPort  ActionType=case
  Out1 : Outport
  wires:
  In1/1 -> Out1/1

== system multilevelinverter1/Subsystem2/If Action Subsystem9 ==
  In1 : Inport
  Action Port : ActionPort  ActionType=case
  Out1 : Outport
  wires:
  In1/1 -> Out1/1

== system multilevelinverter1/Subsystem3/PV Boost Converter1 ==
  Analog Filter Design : dsparch4/Analog Filter Design  method=Butterworth  filttype=Lowpass  N=8  Wlo=30  Whi=80  Rp=2  Rs=40
  Analog Filter Design1 : dsparch4/Analog Filter Design  method=Butterworth  filttype=Lowpass  N=8  Wlo=30  Whi=80  Rp=2  Rs=40
  Current Measurement : powerlib/Measurements/Current Measurement  PhasorSimulation=off  OutputType=Complex  PSBequivalent=0
  Diode : powerlib/Power Electronics/Diode  Ron=0.001  Lon=0  Vf=0.8  IC=0  UseSnubber=off  Rs=500  Cs=250e-9  Measurements=on
  MPPT : Subsystem
  Mosfet : powerlib/Power Electronics/Mosfet  Ron=0.1  Lon=0  Rd=0.01  Vfd=0  IC=0  Rs=1e5  Cs=inf  Measurements=on
  PI CONTOLER : Subsystem
  Relational Operator1 : RelationalOperator  Operator=<=  OutDataTypeStr=boolean
  Repeating Sequence : simulink/Sources/Repeating Sequence  rep_seq_t=[0 0.0001 0.0002]  rep_seq_y=[0 10 0]
  Scope{1..3,8} (4 alike) : Scope
      Scope1 settings: SaveName=ScopeData2
      Scope2 settings: SaveName=ScopeData3
      Scope3 settings: YMin=-20  YMax=100  SaveName=ScopeData12
      Scope8 settings: YMin=31.943  YMax=31.943  SaveName=ScopeData4
  Series RLC Branch : powerlib/Elements/Series RLC Branch  LConnTagsString=__new0  RConnTagsString=__new0  BranchType=L  Resistance=1  Inductance=1e-3  SetiL0=off  InitialCurrent=0  Capacitance=1e-6  Setx0=off  InitialVoltage=0  Measurements=None
  Series RLC Branch1 : powerlib/Elements/Series RLC Branch  LConnTagsString=__new0  RConnTagsString=__new0  BranchType=C  Resistance=1  Inductance=12e-3  SetiL0=off  InitialCurrent=0  Capacitance=2200e-6  Setx0=off  InitialVoltage=0  Measurements=None
  Voltage Measurement1 : powerlib/Measurements/Voltage Measurement  PhasorSimulation=off  OutputType=Complex  PSBequivalent=0
  Voltage Measurement2 : powerlib/Measurements/Voltage Measurement  PhasorSimulation=off  OutputType=Complex  PSBequivalent=0
  + : PMIOPort  Port=1  Side=Right
  - : PMIOPort  Port=2  Side=Right
  Vpv+ : PMIOPort  Tag=PMCPort  Port=3  Side=Left
  Vpv- : PMIOPort  Tag=PMCPort  Port=4  Side=Left
  wires:
  [G] -> Mosfet/1
  Voltage Measurement2/1 -> Analog Filter Design1/1, Scope3/1
  PI CONTOLER/1(Out1) -> [G]
  [A1] -> PI CONTOLER/1(In1)
  Voltage Measurement1/1 -> [A1], Scope8/1
  Current Measurement/1 -> Analog Filter Design/1
  Repeating Sequence/1 -> Relational Operator1/1, Scope2/1
  Relational Operator1/1 -> Scope1/1
  MPPT/1(D) -> Relational Operator1/2
  Analog Filter Design/1 -> MPPT/2(I)
  Analog Filter Design1/1 -> MPPT/1(V)
  connections:
  Series RLC Branch/RConn1 -- Mosfet/LConn1 -- Diode/LConn1
  Vpv-/RConn1 -- Voltage Measurement2/LConn2 -- Mosfet/RConn1 -- -/RConn1 -- Voltage Measurement1/LConn2 -- Series RLC Branch1/RConn1
  Voltage Measurement2/LConn1 -- Current Measurement/RConn1 -- Series RLC Branch/LConn1
  Series RLC Branch1/LConn1 -- +/RConn1 -- Voltage Measurement1/LConn1 -- Diode/RConn1
  Current Measurement/LConn1 -- Vpv+/RConn1

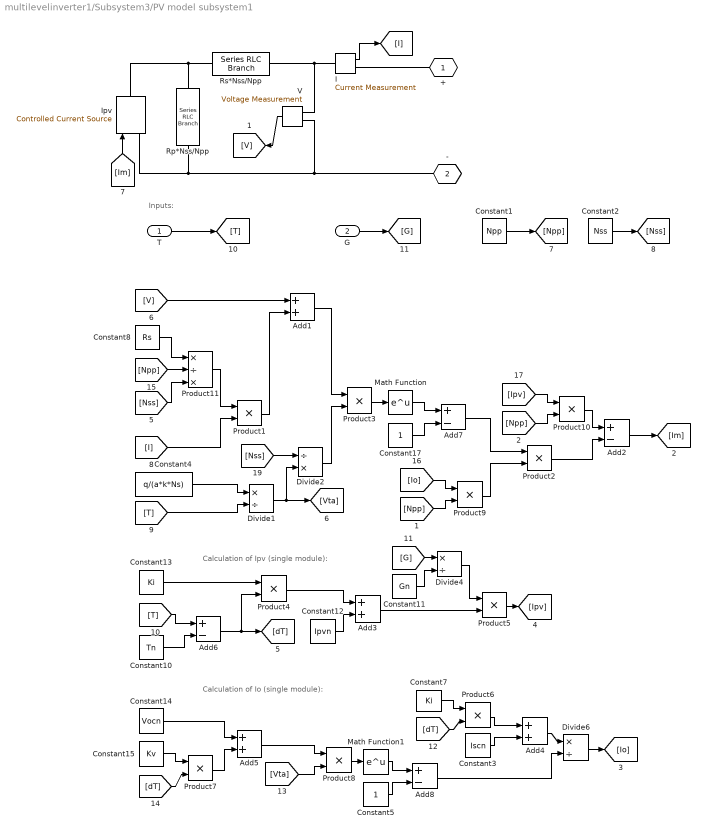
== system multilevelinverter1/Subsystem3/PV model subsystem1 ==
  note: Calculation of Io (single module):
  note: Calculation of Ipv (single module):
  note: Inputs:
  T : Inport
  G : Inport  Port=2
  Add{1,3..5} (4 alike) : Sum
  Add{2,6..8} (4 alike) : Sum  Inputs=+-
  Constant1 : Constant  Value=Npp
  Constant10 : Constant  Value=Tn
  Constant11 : Constant  Value=Gn
  Constant12 : Constant  Value=Ipvn
  Constant13 : Constant  Value=Ki
  Constant14 : Constant  Value=Vocn
  Constant15 : Constant  Value=Kv
  Constant17 : Constant
  Constant2 : Constant  Value=Nss
  Constant3 : Constant  Value=Iscn
  Constant4 : Constant  Value=q/(a*k*Ns)
  Constant5 : Constant
  Constant7 : Constant  Value=Ki
  Constant8 : Constant  Value=Rs
  Divide1 : Product  Inputs=*/
  Divide2 : Product  Inputs=/*
  Divide4 : Product  Inputs=*/
  Divide6 : Product  Inputs=*/
  I : powerlib/Measurements/Current Measurement  PhasorSimulation=off  OutputType=Complex  PSBequivalent=0
  Ipv : powerlib/Electrical Sources/Controlled Current Source  Initialize=on  Source_Type=DC  Amplitude=00  Phase=0  Frequency=0  Measurements=None
  Math Function : Math  SaturateOnIntegerOverflow=on
  Math Function1 : Math  SaturateOnIntegerOverflow=on
  Product{1..10} (10 alike) : Product  RndMeth=Zero
  Product11 : Product  Inputs=*/*  RndMeth=Zero
  Rp*Nss/Npp : powerlib/Elements/Series RLC Branch  LConnTagsString=__new0  RConnTagsString=__new0  BranchType=R  Resistance=Rp*Nss/Npp  Inductance=1e-3  SetiL0=off  InitialCurrent=0  Capacitance=1e-6  Setx0=off  InitialVoltage=0  Measurements=None
  Rs*Nss/Npp : powerlib/Elements/Series RLC Branch  LConnTagsString=__new0  RConnTagsString=__new0  BranchType=R  Resistance=Rs*Nss/Npp  Inductance=1e-3  SetiL0=off  InitialCurrent=0  Capacitance=1e-6  Setx0=off  InitialVoltage=0  Measurements=None
  "V " : powerlib/Measurements/Voltage Measurement  PhasorSimulation=off  OutputType=Complex  PSBequivalent=0
  + : PMIOPort  Port=1  Side=Right
  - : PMIOPort  Port=2  Side=Right
  wires:
  Add4/1 -> Divide6/1
  Add6/1 -> Product4/2, [dT]
  Divide2/1 -> Product3/2
  Divide1/1 -> [Vta], Divide2/2
  [Nss] -> Divide2/1
  Product11/1 -> Product1/1
  [Nss] -> Product11/3
  [Npp] -> Product11/2
  Constant8/1 -> Product11/1
  Product10/1 -> Add2/1
  [Npp] -> Product10/2
  [Ipv] -> Product10/1
  Constant2/1 -> [Nss]
  Constant1/1 -> [Npp]
  [Npp] -> Product9/2
  [Io] -> Product9/1
  Product9/1 -> Product2/2
  Product2/1 -> Add2/2
  Constant12/1 -> Add3/2
  Product6/1 -> Add4/1
  Constant3/1 -> Add4/2
  Add8/1 -> Divide6/2
  [Vta] -> Product8/2
  Constant15/1 -> Product7/1
  Product7/1 -> Add5/2
  Divide4/1 -> Product5/1
  Add3/1 -> Product5/2
  Product4/1 -> Add3/1
  Math Function/1 -> Add7/1
  Product1/1 -> Add1/2
  Product5/1 -> [Ipv]
  Divide6/1 -> [Io]
  Math Function1/1 -> Add8/1
  Constant5/1 -> Add8/2
  Add7/1 -> Product2/1
  Constant17/1 -> Add7/2
  Add5/1 -> Product8/1
  Product8/1 -> Math Function1/1
  Constant14/1 -> Add5/1
  [dT] -> Product7/2
  Constant7/1 -> Product6/1
  [dT] -> Product6/2
  Constant13/1 -> Product4/1
  Constant11/1 -> Divide4/2
  [G] -> Divide4/1
  Add1/1 -> Product3/1
  Add2/1 -> [Im]
  Product3/1 -> Math Function/1
  [V] -> Add1/1
  [T] -> Divide1/2
  Constant4/1 -> Divide1/1
  [I] -> Product1/2
  [T] -> Add6/1
  Constant10/1 -> Add6/2
  T/1 -> [T]
  G/1 -> [G]
  [Im] -> Ipv/1
  "V "/1 -> [V]
  I/1 -> [I]
  connections:
  +/RConn1 -- I/RConn1
  Rp*Nss/Npp/LConn1 -- Rs*Nss/Npp/LConn1 -- Ipv/RConn1
  "V "/LConn2 -- Ipv/LConn1 -- Rp*Nss/Npp/RConn1 -- -/RConn1
  Rs*Nss/Npp/RConn1 -- "V "/LConn1 -- I/LConn1

== system multilevelinverter1/Subsystem4/PV Boost Converter1 ==
  Analog Filter Design : dsparch4/Analog Filter Design  method=Butterworth  filttype=Lowpass  N=8  Wlo=30  Whi=80  Rp=2  Rs=40
  Analog Filter Design1 : dsparch4/Analog Filter Design  method=Butterworth  filttype=Lowpass  N=8  Wlo=30  Whi=80  Rp=2  Rs=40
  Current Measurement : powerlib/Measurements/Current Measurement  PhasorSimulation=off  OutputType=Complex  PSBequivalent=0
  Diode : powerlib/Power Electronics/Diode  Ron=0.001  Lon=0  Vf=0.8  IC=0  UseSnubber=off  Rs=500  Cs=250e-9  Measurements=on
  MPPT : Subsystem
  Mosfet : powerlib/Power Electronics/Mosfet  Ron=0.1  Lon=0  Rd=0.01  Vfd=0  IC=0  Rs=1e5  Cs=inf  Measurements=on
  PI CONTOLER : Subsystem
  Relational Operator1 : RelationalOperator  Operator=<=  OutDataTypeStr=boolean
  Repeating Sequence : simulink/Sources/Repeating Sequence  rep_seq_t=[0 0.0001 0.0002]  rep_seq_y=[0 10 0]
  Scope{1..3,8} (4 alike) : Scope
      Scope1 settings: SaveName=ScopeData2
      Scope2 settings: SaveName=ScopeData3
      Scope3 settings: YMin=-20  YMax=100  SaveName=ScopeData12
      Scope8 settings: YMin=31.943  YMax=31.943  SaveName=ScopeData4
  Series RLC Branch : powerlib/Elements/Series RLC Branch  LConnTagsString=__new0  RConnTagsString=__new0  BranchType=L  Resistance=1  Inductance=1e-3  SetiL0=off  InitialCurrent=0  Capacitance=1e-6  Setx0=off  InitialVoltage=0  Measurements=None
  Series RLC Branch1 : powerlib/Elements/Series RLC Branch  LConnTagsString=__new0  RConnTagsString=__new0  BranchType=C  Resistance=1  Inductance=12e-3  SetiL0=off  InitialCurrent=0  Capacitance=2200e-6  Setx0=off  InitialVoltage=0  Measurements=None
  Voltage Measurement1 : powerlib/Measurements/Voltage Measurement  PhasorSimulation=off  OutputType=Complex  PSBequivalent=0
  Voltage Measurement2 : powerlib/Measurements/Voltage Measurement  PhasorSimulation=off  OutputType=Complex  PSBequivalent=0
  + : PMIOPort  Port=1  Side=Right
  - : PMIOPort  Port=2  Side=Right
  Vpv+ : PMIOPort  Tag=PMCPort  Port=3  Side=Left
  Vpv- : PMIOPort  Tag=PMCPort  Port=4  Side=Left
  wires:
  [G] -> Mosfet/1
  Voltage Measurement2/1 -> Analog Filter Design1/1, Scope3/1
  PI CONTOLER/1(Out1) -> [G]
  [A1] -> PI CONTOLER/1(In1)
  Voltage Measurement1/1 -> [A1], Scope8/1
  Current Measurement/1 -> Analog Filter Design/1
  Repeating Sequence/1 -> Relational Operator1/1, Scope2/1
  Relational Operator1/1 -> Scope1/1
  MPPT/1(D) -> Relational Operator1/2
  Analog Filter Design/1 -> MPPT/2(I)
  Analog Filter Design1/1 -> MPPT/1(V)
  connections:
  Series RLC Branch/RConn1 -- Mosfet/LConn1 -- Diode/LConn1
  Vpv-/RConn1 -- Voltage Measurement2/LConn2 -- Mosfet/RConn1 -- -/RConn1 -- Voltage Measurement1/LConn2 -- Series RLC Branch1/RConn1
  Voltage Measurement2/LConn1 -- Current Measurement/RConn1 -- Series RLC Branch/LConn1
  Series RLC Branch1/LConn1 -- +/RConn1 -- Voltage Measurement1/LConn1 -- Diode/RConn1
  Current Measurement/LConn1 -- Vpv+/RConn1

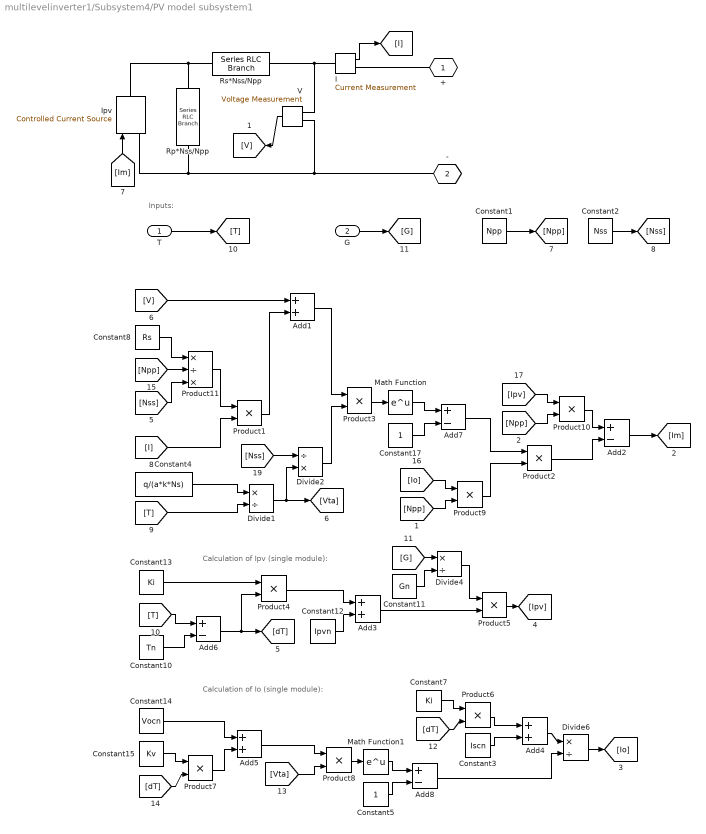
== system multilevelinverter1/Subsystem4/PV model subsystem1 ==
  note: Calculation of Io (single module):
  note: Calculation of Ipv (single module):
  note: Inputs:
  T : Inport
  G : Inport  Port=2
  Add{1,3..5} (4 alike) : Sum
  Add{2,6..8} (4 alike) : Sum  Inputs=+-
  Constant1 : Constant  Value=Npp
  Constant10 : Constant  Value=Tn
  Constant11 : Constant  Value=Gn
  Constant12 : Constant  Value=Ipvn
  Constant13 : Constant  Value=Ki
  Constant14 : Constant  Value=Vocn
  Constant15 : Constant  Value=Kv
  Constant17 : Constant
  Constant2 : Constant  Value=Nss
  Constant3 : Constant  Value=Iscn
  Constant4 : Constant  Value=q/(a*k*Ns)
  Constant5 : Constant
  Constant7 : Constant  Value=Ki
  Constant8 : Constant  Value=Rs
  Divide1 : Product  Inputs=*/
  Divide2 : Product  Inputs=/*
  Divide4 : Product  Inputs=*/
  Divide6 : Product  Inputs=*/
  I : powerlib/Measurements/Current Measurement  PhasorSimulation=off  OutputType=Complex  PSBequivalent=0
  Ipv : powerlib/Electrical Sources/Controlled Current Source  Initialize=on  Source_Type=DC  Amplitude=00  Phase=0  Frequency=0  Measurements=None
  Math Function : Math  SaturateOnIntegerOverflow=on
  Math Function1 : Math  SaturateOnIntegerOverflow=on
  Product{1..10} (10 alike) : Product  RndMeth=Zero
  Product11 : Product  Inputs=*/*  RndMeth=Zero
  Rp*Nss/Npp : powerlib/Elements/Series RLC Branch  LConnTagsString=__new0  RConnTagsString=__new0  BranchType=R  Resistance=Rp*Nss/Npp  Inductance=1e-3  SetiL0=off  InitialCurrent=0  Capacitance=1e-6  Setx0=off  InitialVoltage=0  Measurements=None
  Rs*Nss/Npp : powerlib/Elements/Series RLC Branch  LConnTagsString=__new0  RConnTagsString=__new0  BranchType=R  Resistance=Rs*Nss/Npp  Inductance=1e-3  SetiL0=off  InitialCurrent=0  Capacitance=1e-6  Setx0=off  InitialVoltage=0  Measurements=None
  "V " : powerlib/Measurements/Voltage Measurement  PhasorSimulation=off  OutputType=Complex  PSBequivalent=0
  + : PMIOPort  Port=1  Side=Right
  - : PMIOPort  Port=2  Side=Right
  wires:
  Add4/1 -> Divide6/1
  Add6/1 -> Product4/2, [dT]
  Divide2/1 -> Product3/2
  Divide1/1 -> [Vta], Divide2/2
  [Nss] -> Divide2/1
  Product11/1 -> Product1/1
  [Nss] -> Product11/3
  [Npp] -> Product11/2
  Constant8/1 -> Product11/1
  Product10/1 -> Add2/1
  [Npp] -> Product10/2
  [Ipv] -> Product10/1
  Constant2/1 -> [Nss]
  Constant1/1 -> [Npp]
  [Npp] -> Product9/2
  [Io] -> Product9/1
  Product9/1 -> Product2/2
  Product2/1 -> Add2/2
  Constant12/1 -> Add3/2
  Product6/1 -> Add4/1
  Constant3/1 -> Add4/2
  Add8/1 -> Divide6/2
  [Vta] -> Product8/2
  Constant15/1 -> Product7/1
  Product7/1 -> Add5/2
  Divide4/1 -> Product5/1
  Add3/1 -> Product5/2
  Product4/1 -> Add3/1
  Math Function/1 -> Add7/1
  Product1/1 -> Add1/2
  Product5/1 -> [Ipv]
  Divide6/1 -> [Io]
  Math Function1/1 -> Add8/1
  Constant5/1 -> Add8/2
  Add7/1 -> Product2/1
  Constant17/1 -> Add7/2
  Add5/1 -> Product8/1
  Product8/1 -> Math Function1/1
  Constant14/1 -> Add5/1
  [dT] -> Product7/2
  Constant7/1 -> Product6/1
  [dT] -> Product6/2
  Constant13/1 -> Product4/1
  Constant11/1 -> Divide4/2
  [G] -> Divide4/1
  Add1/1 -> Product3/1
  Add2/1 -> [Im]
  Product3/1 -> Math Function/1
  [V] -> Add1/1
  [T] -> Divide1/2
  Constant4/1 -> Divide1/1
  [I] -> Product1/2
  [T] -> Add6/1
  Constant10/1 -> Add6/2
  T/1 -> [T]
  G/1 -> [G]
  [Im] -> Ipv/1
  "V "/1 -> [V]
  I/1 -> [I]
  connections:
  +/RConn1 -- I/RConn1
  Rp*Nss/Npp/LConn1 -- Rs*Nss/Npp/LConn1 -- Ipv/RConn1
  "V "/LConn2 -- Ipv/LConn1 -- Rp*Nss/Npp/RConn1 -- -/RConn1
  Rs*Nss/Npp/RConn1 -- "V "/LConn1 -- I/LConn1

== system multilevelinverter1/Subsystem5/PV Boost Converter1 ==
  Analog Filter Design : dsparch4/Analog Filter Design  method=Butterworth  filttype=Lowpass  N=8  Wlo=30  Whi=80  Rp=2  Rs=40
  Analog Filter Design1 : dsparch4/Analog Filter Design  method=Butterworth  filttype=Lowpass  N=8  Wlo=30  Whi=80  Rp=2  Rs=40
  Current Measurement : powerlib/Measurements/Current Measurement  PhasorSimulation=off  OutputType=Complex  PSBequivalent=0
  Diode : powerlib/Power Electronics/Diode  Ron=0.001  Lon=0  Vf=0.8  IC=0  UseSnubber=off  Rs=500  Cs=250e-9  Measurements=on
  MPPT : Subsystem
  Mosfet : powerlib/Power Electronics/Mosfet  Ron=0.1  Lon=0  Rd=0.01  Vfd=0  IC=0  Rs=1e5  Cs=inf  Measurements=on
  PI CONTOLER : Subsystem
  Relational Operator1 : RelationalOperator  Operator=<=  OutDataTypeStr=boolean
  Repeating Sequence : simulink/Sources/Repeating Sequence  rep_seq_t=[0 0.0001 0.0002]  rep_seq_y=[0 10 0]
  Scope{1..3,8} (4 alike) : Scope
      Scope1 settings: SaveName=ScopeData2
      Scope2 settings: SaveName=ScopeData3
      Scope3 settings: YMin=-20  YMax=100  SaveName=ScopeData12
      Scope8 settings: YMin=31.943  YMax=31.943  SaveName=ScopeData4
  Series RLC Branch : powerlib/Elements/Series RLC Branch  LConnTagsString=__new0  RConnTagsString=__new0  BranchType=L  Resistance=1  Inductance=1e-3  SetiL0=off  InitialCurrent=0  Capacitance=1e-6  Setx0=off  InitialVoltage=0  Measurements=None
  Series RLC Branch1 : powerlib/Elements/Series RLC Branch  LConnTagsString=__new0  RConnTagsString=__new0  BranchType=C  Resistance=1  Inductance=12e-3  SetiL0=off  InitialCurrent=0  Capacitance=2200e-6  Setx0=off  InitialVoltage=0  Measurements=None
  Voltage Measurement1 : powerlib/Measurements/Voltage Measurement  PhasorSimulation=off  OutputType=Complex  PSBequivalent=0
  Voltage Measurement2 : powerlib/Measurements/Voltage Measurement  PhasorSimulation=off  OutputType=Complex  PSBequivalent=0
  + : PMIOPort  Port=1  Side=Right
  - : PMIOPort  Port=2  Side=Right
  Vpv+ : PMIOPort  Tag=PMCPort  Port=3  Side=Left
  Vpv- : PMIOPort  Tag=PMCPort  Port=4  Side=Left
  wires:
  Analog Filter Design1/1 -> MPPT/1(V)
  Analog Filter Design/1 -> MPPT/2(I)
  MPPT/1(D) -> Relational Operator1/2
  Relational Operator1/1 -> Scope1/1
  Repeating Sequence/1 -> Scope2/1, Relational Operator1/1
  Current Measurement/1 -> Analog Filter Design/1
  Voltage Measurement1/1 -> Scope8/1, [A1]
  [A1] -> PI CONTOLER/1(In1)
  PI CONTOLER/1(Out1) -> [G]
  Voltage Measurement2/1 -> Scope3/1, Analog Filter Design1/1
  [G] -> Mosfet/1
  connections:
  Current Measurement/LConn1 -- Vpv+/RConn1
  Diode/RConn1 -- Voltage Measurement1/LConn1 -- +/RConn1 -- Series RLC Branch1/LConn1
  Series RLC Branch/LConn1 -- Current Measurement/RConn1 -- Voltage Measurement2/LConn1
  Series RLC Branch1/RConn1 -- Voltage Measurement1/LConn2 -- -/RConn1 -- Mosfet/RConn1 -- Voltage Measurement2/LConn2 -- Vpv-/RConn1
  Diode/LConn1 -- Mosfet/LConn1 -- Series RLC Branch/RConn1
